simulink library "Qprod"  (R2014b)
settings: Solver=VariableStepAuto  StartTime=0.0  StopTime=10.0  RelTol=1e-3
settings Model: Creator=y.akisheva  LastModifiedBy=Hp
settings DataIOCC: SaveFormat=Dataset
settings OptimizationCC: UseDivisionForNetSlopeComputation=off  SimCompilerOptimization=off
settings DebuggingCC: SolverPrmCheckMsg=none  FrameProcessingCompatibilityMsg=error  AllowSymbolicDim=off
settings HardwareCC: ProdBitPerPointer=64  ProdLargestAtomicFloat=Float  ProdIntDivRoundTo=Zero  ProdEndianess=LittleEndian  ProdWordSize=64  ProdHWDeviceType=Intel->x86-64 (Windows64)
settings RTWCC: RTWCompilerOptimization=off
settings GRTTargetCC: GeneratePreprocessorConditionals=Use local settings
settings ConfigComp: CovMetricSettings=dw  CovHtmlReporting=on  CovSaveCumulativeToWorkspaceVar=on  CovSaveSingleToWorkspaceVar=on  CovExternalEMLEnable=off

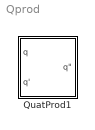
== system Qprod ==
  QuatProd1 : Subsystem  TreatAsAtomicUnit=on
      settings: RTWFcnNameOpts=Use subsystem name  RTWFileNameOpts=Use subsystem name

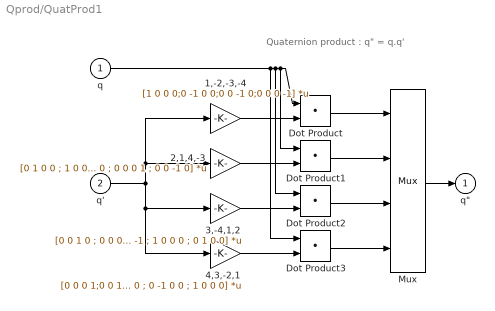
== system Qprod/QuatProd1 ==
  note: Quaternion product : q" = q.q'
  q : Inport  OutDataTypeStr=double  PortDimensions=4
  q' : Inport  Port=2  OutDataTypeStr=double  PortDimensions=4
  1,-2,-3,-4 : Gain  Gain=[1 0 0 0;0 -1 0 0;0 0 -1 0;0 0 0 -1]  Multiplication=Matrix(K*u) (u vector)  SaturateOnIntegerOverflow=on  OutDataTypeStr=Inherit: Same as input  ParamDataTypeStr=Inherit: Same as input
  2,1,4,-3 : Gain  Gain=[0 1 0 0 ; 1 0 0 0 ; 0 0 0 1 ; 0 0 -1 0]  Multiplication=Matrix(K*u) (u vector)  SaturateOnIntegerOverflow=on  OutDataTypeStr=Inherit: Same as input  ParamDataTypeStr=Inherit: Same as input
  3,-4,1,2 : Gain  Gain=[0 0 1 0 ; 0 0 0 -1 ; 1 0 0 0 ; 0 1 0 0]  Multiplication=Matrix(K*u) (u vector)  SaturateOnIntegerOverflow=on  OutDataTypeStr=Inherit: Same as input  ParamDataTypeStr=Inherit: Same as input
  4,3,-2,1 : Gain  Gain=[0 0 0 1;0 0 1 0 ; 0 -1 0 0 ; 1 0 0 0]  Multiplication=Matrix(K*u) (u vector)  SaturateOnIntegerOverflow=on  OutDataTypeStr=Inherit: Same as input  ParamDataTypeStr=Inherit: Same as input
  Dot Product{,1..3} (4 alike) : DotProduct  InputSameDT=on  OutDataTypeStr=Inherit: Inherit via internal rule
  Mux : Mux
  "q\"" : Outport  OutDataTypeStr=double  PortDimensions=4  InitialOutput=0
  wires:
  Mux/1 -> "q\""/1
  Dot Product3/1 -> Mux/4
  Dot Product2/1 -> Mux/3
  Dot Product1/1 -> Mux/2
  Dot Product/1 -> Mux/1
  q/1 -> Dot Product3/1, Dot Product2/1, Dot Product1/1, Dot Product/1
  4,3,-2,1/1 -> Dot Product3/2
  3,-4,1,2/1 -> Dot Product2/2
  2,1,4,-3/1 -> Dot Product1/2
  1,-2,-3,-4/1 -> Dot Product/2
  q'/1 -> 2,1,4,-3/1, 1,-2,-3,-4/1, 4,3,-2,1/1, 3,-4,1,2/1
